simulink model "simulari"  (R2022b)
settings: Solver=VariableStepAuto  StartTime=0.0  StopTime=1000.0  RelTol=1e-3
settings Model: Creator=bogda  LastModifiedBy=bogda

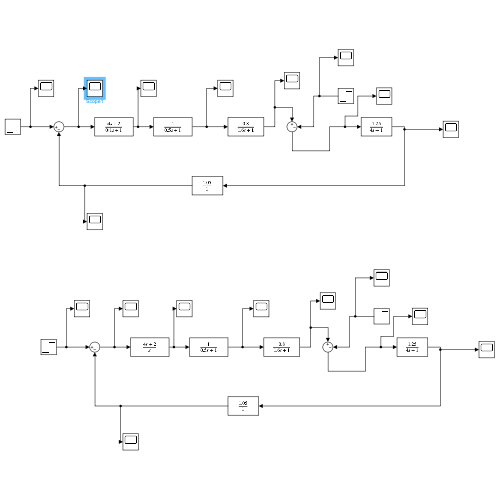
[thumbnail: Simulink's stored preview of the top-level diagram]
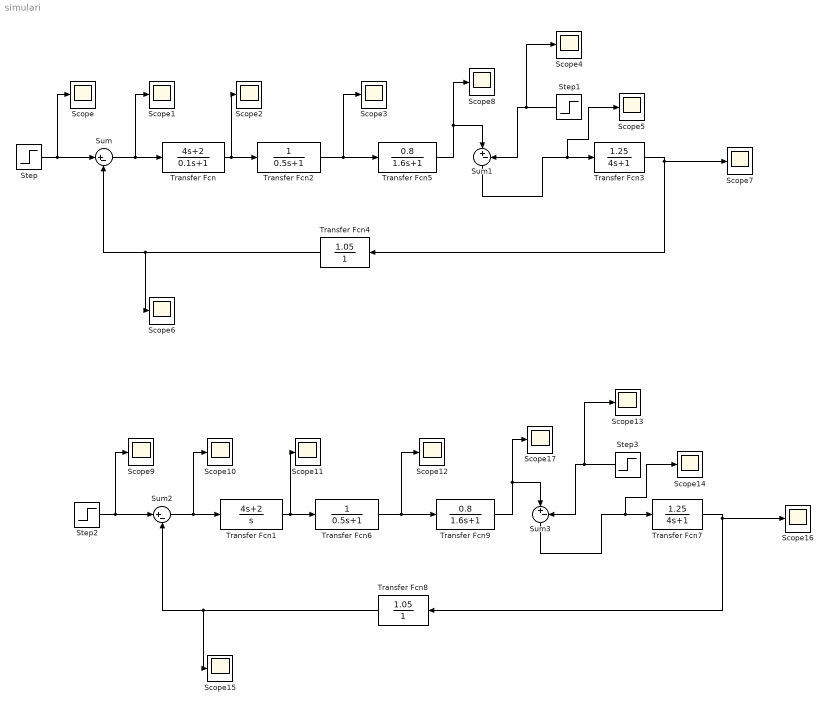
== system simulari ==
  Scope{,1..17} (18 alike) : Scope
  Step : Step  Time=0  After=7  SampleTime=0
  Step1 : Step  Time=400  After=1.25  SampleTime=0
  Step2 : Step  Time=0  After=7  SampleTime=0
  Step3 : Step  Time=400  After=1.25  SampleTime=0
  Sum{,1..3} (4 alike) : Sum  Inputs=|+-
  Transfer Fcn : TransferFcn  Numerator=[4 2]  Denominator=[0.1 1]
  Transfer Fcn1 : TransferFcn  Numerator=[4 2]  Denominator=[1 0]
  Transfer Fcn2 : TransferFcn  Denominator=[0.5 1]
  Transfer Fcn3 : TransferFcn  Numerator=[1.25]  Denominator=[4 1]
  Transfer Fcn4 : TransferFcn  Numerator=[1.05]  Denominator=[1]
  Transfer Fcn5 : TransferFcn  Numerator=[0.8]  Denominator=[1.6 1]
  Transfer Fcn6 : TransferFcn  Denominator=[0.5 1]
  Transfer Fcn7 : TransferFcn  Numerator=[1.25]  Denominator=[4 1]
  Transfer Fcn8 : TransferFcn  Numerator=[1.05]  Denominator=[1]
  Transfer Fcn9 : TransferFcn  Numerator=[0.8]  Denominator=[1.6 1]
  wires:
  Transfer Fcn2/1 -> Transfer Fcn5/1, Scope3/1
  Sum1/1 -> Scope5/1, Transfer Fcn3/1
  Transfer Fcn5/1 -> Scope8/1, Sum1/1
  Step1/1 -> Scope4/1, Sum1/2
  Step/1 -> Scope/1, Sum/1
  Sum/1 -> Scope1/1, Transfer Fcn/1
  Transfer Fcn4/1 -> Scope6/1, Sum/2
  Transfer Fcn/1 -> Transfer Fcn2/1, Scope2/1
  Transfer Fcn3/1 -> Scope7/1, Transfer Fcn4/1
  Transfer Fcn6/1 -> Transfer Fcn9/1, Scope12/1
  Step3/1 -> Scope13/1, Sum3/2
  Sum2/1 -> Scope10/1, Transfer Fcn1/1
  Transfer Fcn9/1 -> Scope17/1, Sum3/1
  Sum3/1 -> Scope14/1, Transfer Fcn7/1
  Step2/1 -> Scope9/1, Sum2/1
  Transfer Fcn1/1 -> Transfer Fcn6/1, Scope11/1
  Transfer Fcn8/1 -> Scope15/1, Sum2/2
  Transfer Fcn7/1 -> Scope16/1, Transfer Fcn8/1
